simulink model "Ziegler_Nichols_open_Loop"  (R2023b)
settings: Solver=ode3  StartTime=0.0  StopTime=50  FixedStep=0.05  RelTol=1e-3  EnableMultiTasking=on
values from neighbouring files (symbols this model uses):
  Vmax = 0.8    [Simulation_code.m]    (also in parameters.m)
  xg = 5    [Simulation_code.m]    (also in parameters.m)
  yg = 5    [Simulation_code.m]    (also in parameters.m)
settings Model: Creator=Shaam  LastModifiedBy=Hadi
settings SolverCC: AlgebraicLoopSolver=TrustRegion
settings DataIOCC: LimitDataPoints=on  SaveFormat=Array  ReturnWorkspaceOutputs=off
settings OptimizationCC: LifeSpan=inf
settings DebuggingCC: UnderspecifiedInitializationDetection=Classic  MergeDetectMultiDrivingBlocksExec=none  SolverPrmCheckMsg=warning  UnconnectedInputMsg=warning  UnconnectedOutputMsg=warning  UnconnectedLineMsg=warning  StateNameClashWarn=warning  SFUnexpectedBacktrackingDiag=warning  SFNoUnconditionalDefaultTransitionDiag=warning  SFExecutionAtInitializationDiag=none  ArithmeticOperatorsInVariantConditions=warning
settings HardwareCC: ProdBitPerPointer=32  ProdBitPerSizeT=32  ProdBitPerPtrDiffT=32  ProdLargestAtomicFloat=None  ProdIntDivRoundTo=Undefined  ProdEndianess=Unspecified  ProdWordSize=32  ProdHWDeviceType=32-bit Generic
settings ModelReferenceCC: PropagateSignalLabelsOutOfModel=off
settings SFSimCC: SimUseLocalCustomCode=off  CustomCodeUndefinedFunction=UseInterfaceOnly
settings RTWCC: RTWUseLocalCustomCode=off
settings CodeAppCC: StateflowObjectComments=on
settings GRTTargetCC: TargetLangStandard=C89/C90 (ANSI)
settings ConfigComp: CovMetricSettings=dw  CovSaveCumulativeToWorkspaceVar=on  CovSaveSingleToWorkspaceVar=on  CovExternalEMLEnable=off

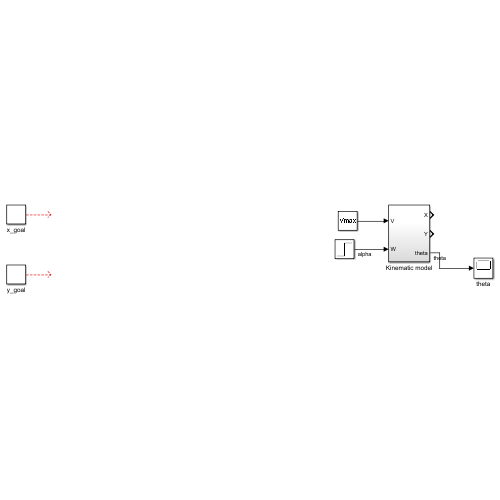
[thumbnail: Simulink's stored preview of the top-level diagram]
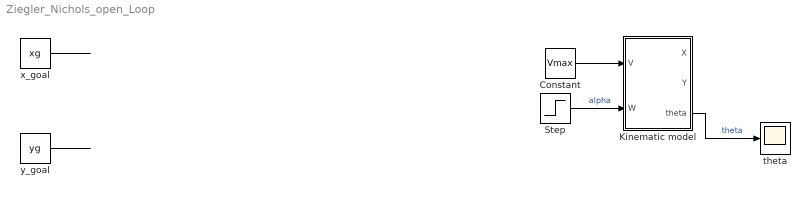
== system Ziegler_Nichols_open_Loop ==
  Constant : Constant  Value=Vmax
  Kinematic model : Subsystem
  Step : Step  Time=0  SampleTime=0
  theta : Scope
  x_goal : Constant  Value=xg
  y_goal : Constant  Value=yg
  wires:
  Kinematic model/3(theta) -> theta/1  "theta"
  x_goal/1 -> ?
  y_goal/1 -> ?
  Constant/1 -> Kinematic model/1(V)
  Step/1 -> Kinematic model/2(W)  "alpha"

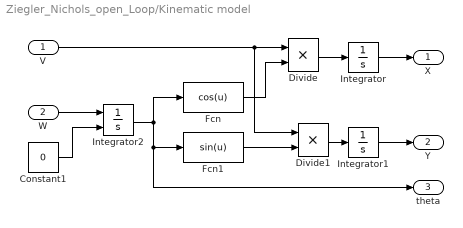
== system Ziegler_Nichols_open_Loop/Kinematic model ==
  V : Inport
  W : Inport  Port=2
  Constant1 : Constant  Value=0
  Divide : Product  Inputs=**
  Divide1 : Product  Inputs=**
  Fcn : Fcn  Expr=cos(u)
  Fcn1 : Fcn  Expr=sin(u)
  Integrator : Integrator
  Integrator1 : Integrator
  Integrator2 : Integrator  InitialConditionSource=external
  X : Outport
  Y : Outport  Port=2
  theta : Outport  Port=3
  wires:
  V/1 -> Divide1/1, Divide/1
  W/1 -> Integrator2/1
  Integrator2/1 -> theta/1, Fcn1/1, Fcn/1
  Divide1/1 -> Integrator1/1
  Fcn/1 -> Divide/2
  Divide/1 -> Integrator/1
  Integrator1/1 -> Y/1
  Integrator/1 -> X/1
  Fcn1/1 -> Divide1/2
  Constant1/1 -> Integrator2/2
